simulink model "model_final_newton"  (R2022a)
settings: Solver=FixedStepAuto  StartTime=0.0  StopTime=10  FixedStep=Auto  RelTol=1e-3
values from neighbouring files (symbols this model uses):
  SS_A = [0 0 1 0;0 0 0 1; 0 G C+D A+B;0 L J I]    [final_init.m]
  SS_B = [0;0;E+F;K]    [final_init.m]
  SS_C = [1 0 0 0;0 1 0 0]    [final_init.m]
  SS_D = [0;0]    [final_init.m]
libraries: fuzblock x1
settings Model: Creator=ziad  LastModifiedBy=USER
settings DebuggingCC: UnconnectedInputMsg=warning  UnconnectedOutputMsg=warning  UnconnectedLineMsg=warning  SFMachineParentedDataDiag=warning
settings RTWCC: DLArmComputeVersion=19.05

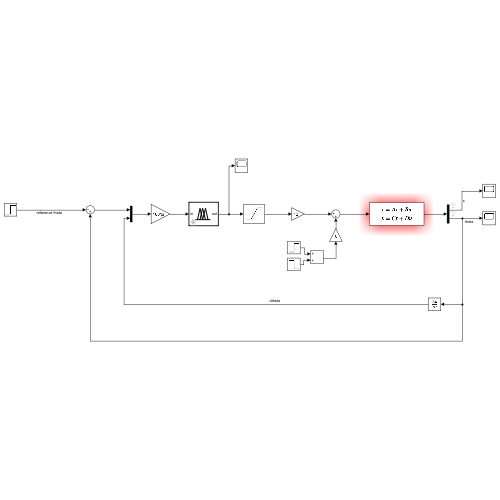
[thumbnail: Simulink's stored preview of the top-level diagram]
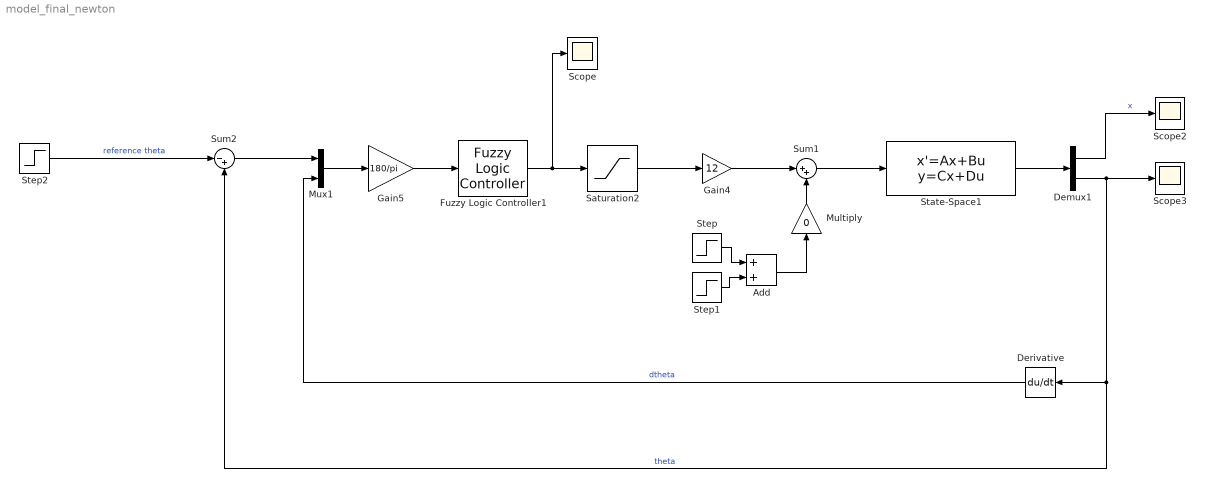
== system model_final_newton ==
  Add : Sum
  Demux1 : Demux  Outputs=2
  Derivative : Derivative
  Fuzzy Logic Controller1 : fuzblock/Fuzzy Logic  Controller  FIS="\"Fuzzy_Logic_Controller_4.fis\""  OutputSampleNumber=101  DataType=double  FuzzifiedInputs=off  RuleFiringStrengths=off  RuleOutputs=off  AggregatedOutputs=off  SimulateUsing=Interpreted execution  OutOfRangeInputValueMessage=warning  NoRuleFiredMessage=warning  EmptyOutputFuzzySetMessage=warning
  Gain4 : Gain  Gain=12
  Gain5 : Gain  Gain=180/pi
  Multiply : Gain  Gain=0
  Mux1 : Mux  Inputs=2
  Saturation2 : Saturate  UpperLimit=1  LowerLimit=-1
  Scope : Scope
  Scope2 : Scope
  Scope3 : Scope
  State-Space1 : StateSpace  A=SS_A  B=SS_B  C=SS_C  D=SS_D  InitialCondition=0
  Step : Step  SampleTime=0
  Step1 : Step  Time=1.026  Before=1  After=0  SampleTime=0
  Step2 : Step  After=0  SampleTime=0
  Sum1 : Sum  Inputs=|++
  Sum2 : Sum  Inputs=|-+
  wires:
  Step/1 -> Add/1
  Step1/1 -> Add/2
  Sum1/1 -> State-Space1/1
  Multiply/1 -> Sum1/2
  Add/1 -> Multiply/1
  State-Space1/1 -> Demux1/1
  Demux1/1 -> Scope2/1  "x"
  Demux1/2 -> Derivative/1, Sum2/2, Scope3/1  "theta"
  Step2/1 -> Sum2/1  "reference theta"
  Sum2/1 -> Mux1/1
  Derivative/1 -> Mux1/2  "dtheta"
  Fuzzy Logic Controller1/1 -> Scope/1, Saturation2/1
  Saturation2/1 -> Gain4/1
  Gain4/1 -> Sum1/1
  Gain5/1 -> Fuzzy Logic Controller1/1
  Mux1/1 -> Gain5/1
